simulink model "mophongsimulink"  (R2018a)
settings: Solver=VariableStepAuto  StartTime=0.0  StopTime=8.5  RelTol=1e-3
libraries: dspsigops x6, simulink x2
settings Model: Creator=Asus  LastModifiedBy=Asus

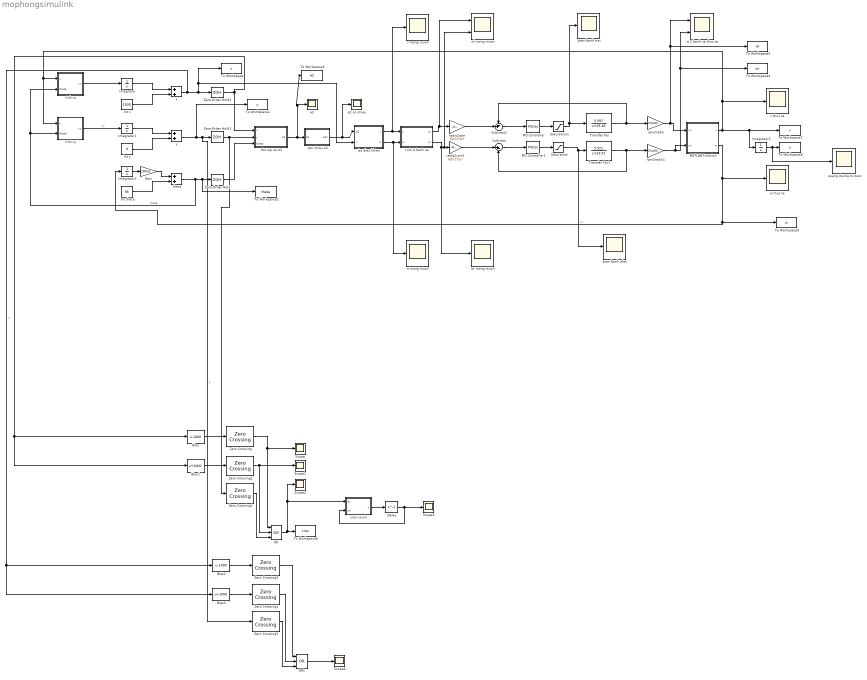
== system mophongsimulink ==
  Bias : Bias  Bias=-1000
  Bias1 : Bias  Bias=1000
  Bias2 : Bias  Bias=-1000
  Bias3 : Bias  Bias=1000
  Delay : Delay  DelayLength=1  SampleTime=0.1
  Gain : Gain  Gain=180/pi
  Int theta : Constant  Value=95
  Int x : Constant  Value=1500
  Int y : Constant  Value=0
  Integrator{,1..3} (4 alike) : Integrator
  MATLAB Function : MATLAB Function  TreatAsAtomicUnit=on
  OR : Logic  Operator=OR  Inputs=3  IconShape=distinctive  AllPortsSameDT=off  OutDataTypeStr=boolean
  OR1 : Logic  Operator=OR  Inputs=3  IconShape=distinctive  AllPortsSameDT=off  OutDataTypeStr=boolean
  PID Controller : simulink/Continuous/PID Controller  Controller=PID  TimeDomain=Continuous-time  SampleTime=-1  IntegratorMethod=Forward Euler  FilterMethod=Forward Euler  Form=Parallel  UseFilter=on  ControllerParametersSource=internal  P=6.1451  I=162.5025  D=0  N=100  InitialConditionSource=internal  InitialConditionForIntegrator=0  InitialConditionForFilter=0  ExternalReset=none  LimitOutput=off  UpperSaturationLimit=inf  LowerSaturationLimit=-inf  LinearizeAsGain=on  AntiWindupMode=none  Kb=1  TrackingMode=off  Kt=1  PParamMin=[]  PParamMax=[]  IParamMin=[]  IParamMax=[]  DParamMin=[]  DParamMax=[]  NParamMin=[]  NParamMax=[]  KbParamMin=[]  KbParamMax=[]  KtParamMin=[]  KtParamMax=[]  POutMin=[]  POutMax=[]  IOutMin=[]  IOutMax=[]  DOutMin=[]  DOutMax=[]  NOutMin=[]  NOutMax=[]  KbOutMin=[]  KbOutMax=[]  KtOutMin=[]  KtOutMax=[]  IntegratorOutMin=[]  IntegratorOutMax=[]  FilterOutMin=[]  FilterOutMax=[]  SumOutMin=[]  SumOutMax=[]  SumI1OutMin=[]  SumI1OutMax=[]  SumI2OutMin=[]  SumI2OutMax=[]  SumI3OutMin=[]  SumI3OutMax=[]  SumDOutMin=[]  SumDOutMax=[]  SaturationOutMin=[]  SaturationOutMax=[]  IntegratorContinuousStateAttributes=''  IntegratorStateMustResolveToSignalObject=off  IntegratorRTWStateStorageClass=Auto  FilterContinuousStateAttributes=''  FilterStateMustResolveToSignalObject=off  FilterRTWStateStorageClass=Auto  DifferentiatorICPrevScaledInput=0  DifferentiatorOutMin=[]  DifferentiatorOutMax=[]  FilterDiffOutCoefMin=[]  FilterDiffOutCoefMax=[]  SumDenOutMin=[]  SumDenOutMax=[]  SumNumOutMin=[]  SumNumOutMax=[]  ReciprocalOutMin=[]  ReciprocalOutMax=[]  DivideOutMin=[]  DivideOutMax=[]  TunerSelectOption=Transfer Function Based (PID Tuner App)
  PID Controller1 : simulink/Continuous/PID Controller  Controller=PID  TimeDomain=Continuous-time  SampleTime=-1  IntegratorMethod=Forward Euler  FilterMethod=Forward Euler  Form=Parallel  UseFilter=on  ControllerParametersSource=internal  P=5.2531  I=144.4473  D=0  N=100  InitialConditionSource=internal  InitialConditionForIntegrator=0  InitialConditionForFilter=0  ExternalReset=none  LimitOutput=off  UpperSaturationLimit=inf  LowerSaturationLimit=-inf  LinearizeAsGain=on  AntiWindupMode=none  Kb=1  TrackingMode=off  Kt=1  PParamMin=[]  PParamMax=[]  IParamMin=[]  IParamMax=[]  DParamMin=[]  DParamMax=[]  NParamMin=[]  NParamMax=[]  KbParamMin=[]  KbParamMax=[]  KtParamMin=[]  KtParamMax=[]  POutMin=[]  POutMax=[]  IOutMin=[]  IOutMax=[]  DOutMin=[]  DOutMax=[]  NOutMin=[]  NOutMax=[]  KbOutMin=[]  KbOutMax=[]  KtOutMin=[]  KtOutMax=[]  IntegratorOutMin=[]  IntegratorOutMax=[]  FilterOutMin=[]  FilterOutMax=[]  SumOutMin=[]  SumOutMax=[]  SumI1OutMin=[]  SumI1OutMax=[]  SumI2OutMin=[]  SumI2OutMax=[]  SumI3OutMin=[]  SumI3OutMax=[]  SumDOutMin=[]  SumDOutMax=[]  SaturationOutMin=[]  SaturationOutMax=[]  IntegratorContinuousStateAttributes=''  IntegratorStateMustResolveToSignalObject=off  IntegratorRTWStateStorageClass=Auto  FilterContinuousStateAttributes=''  FilterStateMustResolveToSignalObject=off  FilterRTWStateStorageClass=Auto  DifferentiatorICPrevScaledInput=0  DifferentiatorOutMin=[]  DifferentiatorOutMax=[]  FilterDiffOutCoefMin=[]  FilterDiffOutCoefMax=[]  SumDenOutMin=[]  SumDenOutMax=[]  SumNumOutMin=[]  SumNumOutMax=[]  ReciprocalOutMin=[]  ReciprocalOutMax=[]  DivideOutMin=[]  DivideOutMax=[]  TunerSelectOption=Transfer Function Based (PID Tuner App)
  Saturation : Saturate  UpperLimit=1000  LowerLimit=0
  Saturation1 : Saturate  UpperLimit=1000  LowerLimit=0
  Scope{,1..4} (5 alike) : Scope
  Subtract : Sum  Inputs=|+-
  Subtract1 : Sum  Inputs=-+|
  To Workspace : ToWorkspace  VariableName=x  SampleTime=0.1
  To Workspace1 : ToWorkspace  VariableName=y  SampleTime=0.1
  To Workspace2 : ToWorkspace  VariableName=theta  SampleTime=0.1
  To Workspace3 : ToWorkspace  VariableName=e2  SampleTime=0.1
  To Workspace4 : ToWorkspace  VariableName=wr  SampleTime=0.1
  To Workspace5 : ToWorkspace  VariableName=wl  SampleTime=0.1
  To Workspace6 : ToWorkspace  VariableName=cros  SampleTime=-1
  To Workspace7 : ToWorkspace  VariableName=v  SampleTime=0.1
  To Workspace8 : ToWorkspace  VariableName=s  SampleTime=0.1
  To Workspace9 : ToWorkspace  VariableName=w  SampleTime=0.1
  Transfer Fcn : TransferFcn  Numerator=[5.597]  Denominator=[1 25.48]
  Transfer Fcn1 : TransferFcn  Numerator=[5.521]  Denominator=[1 23.51]
  Zero Crossing{,1..5} (6 alike) : dspsigops/Zero Crossing  InputProcessing=Columns as channels (frame based)
      settings: SourceProductName=DSP System Toolbox  SourceProductBaseCode=DS
  Zero-Order Hold : ZeroOrderHold  SampleTime=0.1
  Zero-Order Hold1 : ZeroOrderHold  SampleTime=0.1
  Zero-Order Hold2 : ZeroOrderHold  SampleTime=0.1
  bo dieu khien : MATLAB Function  TreatAsAtomicUnit=on
  cros count : MATLAB Function  TreatAsAtomicUnit=on
  doc sai so e2 : MATLAB Function  TreatAsAtomicUnit=on
  e2 : Scope
  e2 co nhieu : Scope
  pwm banh phai : Scope
  pwm banh trai : Scope
  quang duong di duoc : Scope
  rad/s2rpm : Gain  Gain=60/(2*pi)
  rad/s2rpm1 : Gain  Gain=60/(2*pi)
  rpm2rad/s : Gain  Gain=2*pi/60
  rpm2rad/s1 : Gain  Gain=2*pi/60
  "tao nhieu e2 " : MATLAB Function  TreatAsAtomicUnit=on
  theta : Sum
  tinh vx : MATLAB Function  TreatAsAtomicUnit=on
  tinh vy : MATLAB Function  TreatAsAtomicUnit=on
  tinh w banh xe : MATLAB Function  TreatAsAtomicUnit=on
  v mong muon : Scope
  v thuc te : Scope
  w 2 banh xe thuc te : Scope  NumInputPorts=2
  w mong muon : Scope
  w thuc te : Scope
  wl mong muon : Scope  NumInputPorts=2
  wr mong muon : Scope
  x : Sum
  y : Sum
  wires:
  Int x/1 -> x/2
  Integrator/1 -> x/1
  x/1 -> Bias2/1, Bias3/1, bo dieu khien/2(x), To Workspace/1, Zero-Order Hold2/1  "x"
  Int y/1 -> y/2
  y/1 -> To Workspace1/1, Zero Crossing5/1, Zero-Order Hold1/1  "y"
  tinh vy/1(vy) -> Integrator1/1  "vy"
  Integrator1/1 -> y/1
  theta/1 -> To Workspace2/1, Zero-Order Hold/1, tinh vy/2(theta), tinh vx/2(theta)  "theta"
  MATLAB Function/2(w) -> w thuc te/1, To Workspace9/1, Integrator2/1  "w"
  Int theta/1 -> theta/2
  Integrator2/1 -> Gain/1
  Gain/1 -> theta/1
  doc sai so e2/1(e2) -> To Workspace3/1, e2/1, "tao nhieu e2 "/1(e2)
  bo dieu khien/1(v) -> v mong muon/1, tinh w banh xe/1(v)
  tinh w banh xe/2(wr) -> wr mong muon/1, wl mong muon/2, rad/s2rpm1/1
  tinh w banh xe/1(wl) -> wl mong muon/1, rad/s2rpm/1
  Subtract/1 -> PID Controller1/1
  Subtract1/1 -> PID Controller/1
  PID Controller1/1 -> Saturation/1
  PID Controller/1 -> Saturation1/1
  Transfer Fcn/1 -> rpm2rad/s/1, Subtract1/1
  Transfer Fcn1/1 -> rpm2rad/s1/1, Subtract/2
  rpm2rad/s/1 -> To Workspace5/1, w 2 banh xe thuc te/1, MATLAB Function/1(wl)
  rpm2rad/s1/1 -> To Workspace4/1, w 2 banh xe thuc te/2, MATLAB Function/2(wr)
  tinh vx/1(vx) -> Integrator/1
  Zero-Order Hold/1 -> doc sai so e2/3(theta)
  Zero-Order Hold1/1 -> Zero Crossing2/1, doc sai so e2/2(y)
  Zero-Order Hold2/1 -> doc sai so e2/1(x), Bias1/1, Bias/1
  MATLAB Function/1(v) -> v thuc te/1, tinh vx/1(v), tinh vy/1(v), Integrator3/1, To Workspace7/1
  bo dieu khien/2(w) -> w mong muon/1, tinh w banh xe/2(w)
  "tao nhieu e2 "/1(e2n) -> e2 co nhieu/1, bo dieu khien/1(e2)
  Saturation/1 -> pwm banh phai/1, Transfer Fcn1/1
  rad/s2rpm/1 -> Subtract1/2
  rad/s2rpm1/1 -> Subtract/1
  Bias/1 -> Zero Crossing/1
  Bias1/1 -> Zero Crossing1/1
  Zero Crossing/1 -> Scope/1, OR/1
  Zero Crossing1/1 -> Scope1/1, OR/2
  OR/1 -> cros count/1(dt), Scope2/1, To Workspace6/1
  Integrator3/1 -> quang duong di duoc/1, To Workspace8/1
  Zero Crossing2/1 -> OR/3
  cros count/1(y) -> Delay/1
  Delay/1 -> Scope3/1, cros count/2(yo)
  Saturation1/1 -> pwm banh trai/1, Transfer Fcn/1
  Bias3/1 -> Zero Crossing4/1
  Zero Crossing5/1 -> OR1/3
  Zero Crossing3/1 -> OR1/1
  Zero Crossing4/1 -> OR1/2
  Bias2/1 -> Zero Crossing3/1
  OR1/1 -> Scope4/1

== matlab function mophongsimulink/bo dieu khien ==
  data: e2 input; v output; w output; x input
function [v,w]=bodieukhien(e2,x)
%if(x>1000||x<-1000)
   % if(abs(e2)<60)
    v=800;
    w=e2*0.045;
   % else
   %     v=0;
   %     w=0;
   % end
%else
%   if(x>0)
%   v=(1000-x)/10+800;
%    else
%    v=(1000+x)/10+800;
%    end
%w=e2*0.045;    
%end
%end

== matlab function mophongsimulink/doc sai so e2 ==
  data: x input; e2 output; y input; theta input
function e2=docsaisoe2(x,y,theta)
Dc=257;
out=-1;
ssx=x+Dc*cosd(theta);
ssy=y+Dc*sind(theta);  
sstheta=theta+90;  % Toa do cua day cam bien
 r=-ssx*sind(sstheta)+ssy*cosd(sstheta); %tim phuong trinh duong sensor
 check=1;
 e2=-1;                      
 A=[-sind(sstheta) cosd(sstheta); 0 1];   %phuong trinh duong line duoi
 B= [r ; -500];
 temp=A\B;
 xR=temp(1);
 yR=temp(2);
 if(isinf(xR)==0&&isinf(yR)==0&&isnan(xR)==0&&isnan(yR)==0)
     if((xR>-1000)&&(xR<1000))
         e2fake=sqrt((xR-ssx)^2+(yR-ssy)^2);
         if (check==1||e2fake<e2)
             if(ssy<yR)
             out=1;
             else
              out=0;
             end
            e2=e2fake;
            check=0;
         end
     end
 end
 A=[-sind(sstheta) cosd(sstheta); 0 1];   %phuong trinh duong line tren
 B= [r ; 500];
 temp=A\B;
 xR=temp(1);
 yR=temp(2);
 if(isinf(xR)==0&&isinf(yR)==0&&isnan(xR)==0&&isnan(yR)==0)
      if(xR>-1000&&xR<1000)
         e2fake=sqrt((xR-ssx)^2+(yR-ssy)^2);
          if (check==1||e2fake<e2)
              if(ssy>yR)
             out=1;
             else
              out=0;
             end
              e2=e2fake;
              check=0;
          end
      end
 end              
if(abs(cosd(sstheta))<0.001)                        %phuong trinh duong line phai
   xR1=r/(-sind(sstheta)); 
   xR2=r/(-sind(sstheta)); 
   if(250000-(xR1-1000)^2>=0)
     yR1=sqrt(250000-(xR1-1000)^2);
     yR2=-sqrt(250000-(xR1-1000)^2);
   else
     xR1=0;
     xR2=0;
     yR1=0;
     yR2=0;
   end
else
    p=[1+tand(sstheta)^2 2*r*tand(sstheta)/cosd(sstheta)-2000 750000+(r/cosd(sstheta))^2];
    temp=roots(p);
    if(imag(temp(1))==0&&imag(temp(2))==0)
    tempt1=real(temp(1));
    tempt2=real(temp(2));
    xR1=tempt1;
    xR2=tempt2;
    yR1=(r+sind(sstheta)*xR1)/cosd(sstheta);
    yR2=(r+sind(sstheta)*xR2)/cosd(sstheta);
    else
    xR1=0;
    yR1=0;
    xR2=0;
    yR2=0;
    end
end
     if(xR1>=1000&&imag(xR1)==0&&imag(yR1)==0)
        e2fake=sqrt((xR1-ssx)^2+(yR1-ssy)^2);
         if (check==1||e2fake<e2)
            if((ssx-1000)^2+ssy^2>250000)
            out=1;
            else
            out=0;
            end
            e2=e2fake;
            check=0;
         end
     end
     if(xR2>=1000&&imag(xR2)==0&&imag(yR2)==0)
        e2fake=sqrt((xR2-ssx)^2+(yR2-ssy)^2);
         if (check==1||e2fake<e2)
            if((ssx-1000)^2+ssy^2>250000)
            out=1;
            else
            out=0;
            end
            e2=e2fake;
            check=0;
         end
     end
 if(abs(cosd(sstheta))<0.001)                        %phuong trinh duong line trai
   xR1=r/(-sind(sstheta)); 
   xR2=r/(-sind(sstheta)); 
   if(250000-(xR(1)+1000)^2>=0)
     yR1=sqrt(250000-(xR1+1000)^2);
     yR2=-sqrt(250000-(xR1+1000)^2);
   else
     xR1=0;
     xR2=0;
     yR1=0;
     yR2=0;
   end
else
    p=[1+tand(sstheta)^2 2*r*tand(sstheta)/cosd(sstheta)+2000 750000+(r/cosd(sstheta))^2];
    temp=roots(p);
    if(imag(temp(1))==0&&imag(temp(2))==0)
    tempt1=real(temp(1));
    tempt2=real(temp(2));
    xR1=tempt1;
    xR2=tempt2;
    yR1=(r+sind(sstheta)*xR1)/cosd(sstheta);
    yR2=(r+sind(sstheta)*xR2)/cosd(sstheta);
    else
    xR1=0;
    yR1=0;
    xR2=0;
    yR2=0;
    end
end
     if(xR1<= -1000&&imag(xR1)==0&&imag(yR1)==0)
        e2fake=sqrt((xR1-ssx)^2+(yR1-ssy)^2);
         if (check==1||e2fake<e2)
             if((ssx+1000)^2+ssy^2>250000)
            out=1;
            else
            out=0;
            end
            e2=e2fake;
            check=0;
         end
     end
     if(xR2<= -1000&&imag(xR2)==0&&imag(yR2)==0)
        e2fake=sqrt((xR2-ssx)^2+(yR2-ssy)^2);
         if (check==1||e2fake<e2)
             if((ssx+1000)^2+ssy^2>250000)
            out=1;
            else
            out=0;
            end
            e2=e2fake;
         end
     end
   e2=e2*(-1)^(out+1);
   e2=double(e2);
end

== matlab function mophongsimulink/tinh w banh xe ==
  data: v input; wl output; w input; wr output
function [wl,wr] = tinhwbanhxe(v,w)
r=40;
L=177;
wl=(v-w*L/2)/r;
wr=(v+w*L/2)/r;
end

== matlab function mophongsimulink/MATLAB Function ==
  data: wl input; v output; wr input; w output
function [v,w] = wtov(wl,wr)
r=40;
b=88.5;
v=(wl+wr)*r/2;
w=(wr-wl)*r/(2*b);

== matlab function mophongsimulink/tinh vx ==
  data: v input; vx output; theta input
function vx = calvx(v,theta)
vx=v*cosd(theta);

== matlab function mophongsimulink/tinh vy ==
  data: v input; vy output; theta input
function vy = calvy(v,theta)
vy=v*sind(theta);

== matlab function mophongsimulink/tao nhieu e2  ==
  data: e2 input; e2n output
function e2n = taonhieue2(e2)

e2n= e2+rand(1)*10-5;

== matlab function mophongsimulink/cros count ==
  data: dt input; y output; yo input
function y = fcn(dt,yo)

if(dt==1)
    y=yo+1;
else
    y=yo;
end
